simulink library "ksplib"  (R2020b)
settings: Solver=VariableStepAuto  StartTime=0.0  StopTime=10.0  RelTol=1e-3
undefined symbols (not defined in the file): kspTxIn0
settings Model: Creator=brianhannan  LastModifiedBy=bhannan

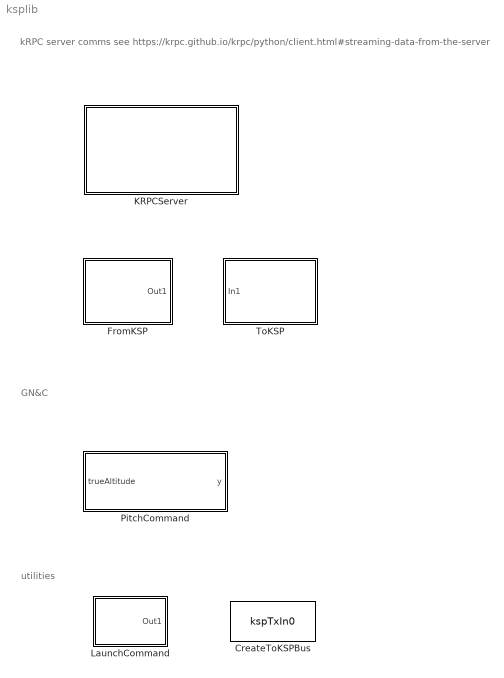
== system ksplib ==
  note: utilities
  note: kRPC server comms
      | see https://krpc.github.io/krpc/python/client.html#streaming-data-from-the-server
  note: GN&C
  CreateToKSPBus : Constant  Value=kspTxIn0  OutDataTypeStr=Bus: kspTxIn
  FromKSP : Subsystem  mask(FromKSP){}
      mask help:
      | Receive data from KSP via kRPC server.
      |
      | This block must be placed in a model with a KRPCServer and a ToKSP block.
      |
      | Outputs a kspRxOut bus. See kspcdemo.sldd, ksp.bus.getRxOutput().
      mask init:
      | ksp.blocks.fromksp.maskInitCbk(gcs);
      mask Display: disp('From KSP')
  KRPCServer : Subsystem  mask(KRPCServer){}
      mask help:
      | Creates a kRPC server instance.
      |
      | This block must be placed in a model with a FromKSP and a ToKSP block.
      mask init:
      | ksp.blocks.krpcserver.maskInitCbk(gcs);
      mask Display: disp('kRPC Server')
  LaunchCommand : Subsystem  mask(Launch Command){launchCmd=logical(0)}
      mask prompts: launchCmd "Launch:"
      mask help: Send launch command
      mask Display: disp('Launch')
  PitchCommand : MATLAB Function  TreatAsAtomicUnit=on  mask(Pitch Command){altitudeVals=[1000, 1800, 6500, 13500, 18500, 31500, 40000], pitchVals=[90, 70, 60, 50, 40, 20, 15]}
      mask prompts: altitudeVals "Altitude (m):"; pitchVals "Pitch (deg):"
      mask help:
      | Calculate pitch command. Provide altitude and pitch values to specify a desired altitude-pitch profile.
      |
      | Input a vector of altitude values (in meters) and a vector of pitch values (a value in degrees between -90 and 90). The output pitch P (deg) is calculated by interpolation using the provided altitude and pitch values and the input altitude (m).
      mask init:
      | altitudePitchEqualLen = numel(altitudeVals) == numel(pitchVals);
      | if ~altitudePitchEqualLen
      |     error(['Altitude and pitch arrays must have the same ' ...
      |         'number of elements.']);
      | end
      | altitudePitchVals = [altitudeVals', pitchVals'];
  ToKSP : Subsystem  mask(ToKSP){}
      mask help:
      | Send data to KSP via kRPC server.
      |
      | This block must be placed in a model with a KRPCServer and a FromKSP block.
      |
      | Input must be a kspTxIn bus. See kspdemo.sldd, ksp.bus.getTxInput().
      mask init:
      | ksp.blocks.toksp.maskInitCbk(gcs);
      mask Display: disp('To KSP')

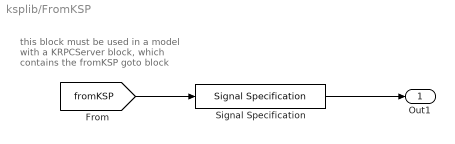
== system ksplib/FromKSP ==
  note: this block must be used in a model with a KRPCServer block, which contains the fromKSP goto block
  Signal Specification : SignalSpecification  OutDataTypeStr=Bus: kspRxOut  BusOutputAsStruct=on
  Out1 : Outport
  wires:
  Signal Specification/1 -> Out1/1
  [fromKSP] -> Signal Specification/1

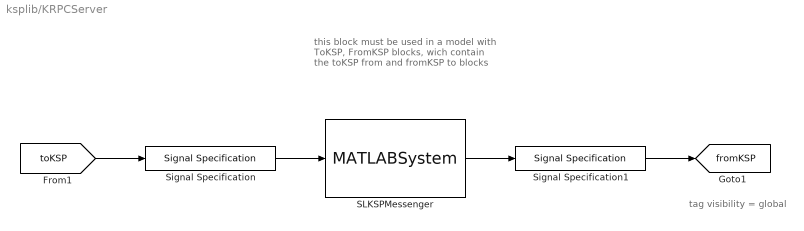
== system ksplib/KRPCServer ==
  note: tag visibility = global
  note: this block must be used in a model with ToKSP, FromKSP blocks, wich contain the toKSP from and fromKSP to blocks
  SLKSPMessenger : MATLABSystem  System=ksp.SLKSPMessenger  SimulateUsing=Interpreted execution
      mask Type: ksp.SLKSPMessenger
      mask Display:
      | disp('KSP TX/RX');
      | port_label('input',1,'u');
      | port_label('output',1,'y');
  Signal Specification : SignalSpecification  OutDataTypeStr=Bus: kspTxIn  BusOutputAsStruct=on
  Signal Specification1 : SignalSpecification  OutDataTypeStr=Bus: kspRxOut  BusOutputAsStruct=on
  tag scope: fromKSP=global
  wires:
  SLKSPMessenger/1 -> Signal Specification1/1
  [toKSP] -> Signal Specification/1
  Signal Specification/1 -> SLKSPMessenger/1
  Signal Specification1/1 -> [fromKSP]

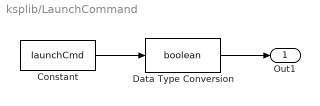
== system ksplib/LaunchCommand ==
  Constant : Constant  Value=launchCmd
  Data Type Conversion : DataTypeConversion  OutDataTypeStr=boolean
  Out1 : Outport
  wires:
  Constant/1 -> Data Type Conversion/1
  Data Type Conversion/1 -> Out1/1

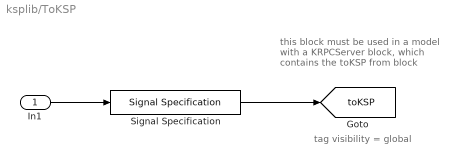
== system ksplib/ToKSP ==
  note: tag visibility = global
  note: this block must be used in a model with a KRPCServer block, which contains the toKSP from block
  In1 : Inport
  Signal Specification : SignalSpecification  OutDataTypeStr=Bus: kspTxIn  BusOutputAsStruct=on
  tag scope: toKSP=global
  wires:
  In1/1 -> Signal Specification/1
  Signal Specification/1 -> [toKSP]

== matlab function ksplib/PitchCommand ==
  data: trueAltitude input double; y output double [-90..90]; altitudePitchVals parameter
function y = calcPitchCommand(trueAltitude, altitudePitchVals)
%CALCPITCHCOMMAND Calculate pitch command (deg.).

validateattributes(trueAltitude,{'double'},{'scalar'})
validateattributes(altitudePitchVals,{'numeric'},{'2d','ncols',2})

altitude0 = altitudePitchVals(:,1);
pitch0 = altitudePitchVals(:,2);
y = interp1(altitude0,pitch0,trueAltitude);
if trueAltitude <= altitude0(1)
    y = pitch0(1);
elseif trueAltitude >= altitude0(end)
    y = pitch0(end);
end

end
